simulink model "ThreeLinkCyl"  (Simulink 7.6)
settings: Solver=ode45  StartTime=0.0  StopTime=10.0  RelTol=1e-3
libraries: roblocks x3, simulink x1
settings Model: Creator=mahyar  LastModifiedBy=mahyar

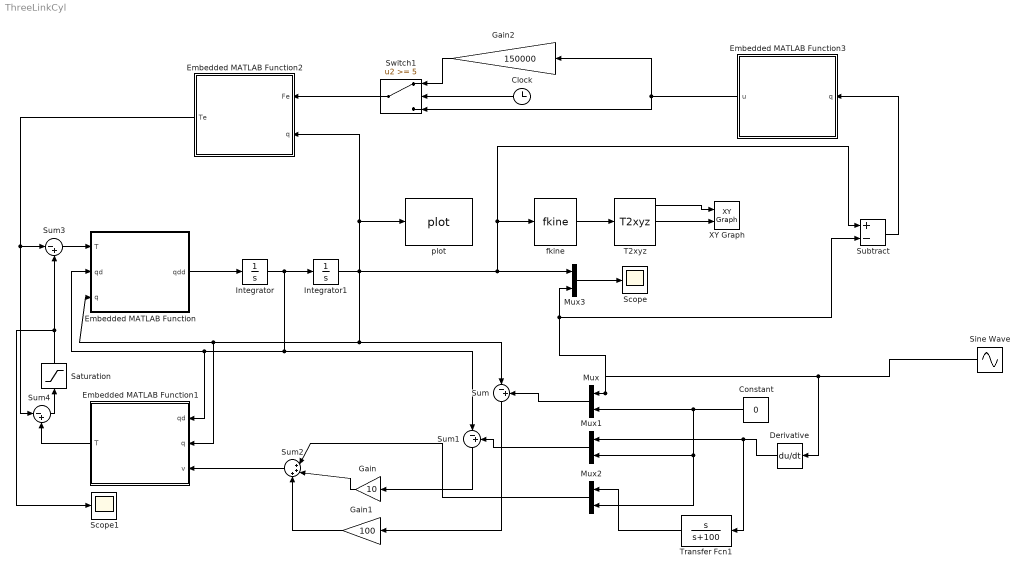
== system ThreeLinkCyl ==
  Clock : Clock
      settings: Decimation=10
  Constant : Constant  Value=0
  Derivative : Derivative
  Embedded MATLAB Function : Stateflow chart  TreatAsAtomicUnit=on
  Embedded MATLAB Function1 : Stateflow chart  TreatAsAtomicUnit=on
  Embedded MATLAB Function2 : Stateflow chart  TreatAsAtomicUnit=on
  Embedded MATLAB Function3 : Stateflow chart  TreatAsAtomicUnit=on
  Gain : Gain  Gain=10
  Gain1 : Gain  Gain=100
  Gain2 : Gain  Gain=150000
  Integrator : Integrator  InitialCondition=[0 0]
  Integrator1 : Integrator  InitialCondition=[0 0]
  Mux{,1..3} (4 alike) : Mux  Inputs=2
  Saturation : Saturate  UpperLimit=85  LowerLimit=-85
  Scope : Scope
      settings: YMin=-1  YMax=1
  Scope1 : Scope
      settings: YMin=-100  YMax=100
  Sine Wave : Sin  SampleTime=0
  Subtract : Sum  Inputs=+-
  Sum{,1,3..4} (4 alike) : Sum  Inputs=|-+
  Sum2 : Sum  Inputs=|+++
  Switch1 : Switch  Threshold=5
  T2xyz : roblocks/T2xyz  SystemSampleTime=-1
  Transfer Fcn1 : TransferFcn  Numerator=[1 0]  Denominator=[1 100]
  XY Graph : simulink/Sinks/XY Graph  SystemSampleTime=-1  xmin=-2  xmax=2  ymin=-2  ymax=2  st=-1
  fkine : roblocks/fkine  SystemSampleTime=-1  robot=tl
  plot : roblocks/plot  SystemSampleTime=-1  robot=tl
  wires:
  Embedded MATLAB Function/1(qdd) -> Integrator/1
  Integrator/1 -> Integrator1/1, Embedded MATLAB Function/2(qd), Embedded MATLAB Function1/1(qd), Sum1/1
  Integrator1/1 -> Embedded MATLAB Function/3(q), Embedded MATLAB Function1/2(q), Sum/1, Mux3/1, fkine/1, Subtract/1, plot/1, Embedded MATLAB Function2/2(q)
  Gain1/1 -> Sum2/3
  Gain/1 -> Sum2/2
  Sum1/1 -> Gain/1
  Sum/1 -> Gain1/1
  Sum2/1 -> Embedded MATLAB Function1/3(v)
  Mux/1 -> Sum/2
  Mux1/1 -> Sum1/2
  Mux2/1 -> Sum2/1
  Derivative/1 -> Mux1/1, Transfer Fcn1/1
  Mux3/1 -> Scope/1
  fkine/1 -> T2xyz/1
  T2xyz/1 -> XY Graph/1
  T2xyz/2 -> XY Graph/2
  Constant/1 -> Mux1/2, Mux2/2, Mux/2
  Embedded MATLAB Function1/1(T) -> Sum4/2
  Sum3/1 -> Embedded MATLAB Function/1(T)
  Subtract/1 -> Embedded MATLAB Function3/1(q)
  Switch1/1 -> Embedded MATLAB Function2/1(Fe)
  Gain2/1 -> Switch1/1
  Embedded MATLAB Function3/1(u) -> Gain2/1, Switch1/3
  Clock/1 -> Switch1/2
  Embedded MATLAB Function2/1(Te) -> Sum3/1, Sum4/1
  Saturation/1 -> Sum3/2, Scope1/1
  Sum4/1 -> Saturation/1
  Transfer Fcn1/1 -> Mux2/1
  Sine Wave/1 -> Mux3/2, Subtract/2, Mux/1, Derivative/1

== matlab function Embedded MATLAB Function1 ==
  data: T output double; qd input double; q input double; v input double
function T = fcn(qd,q,v)

q = [ 0 ; 0 ];
qd = [0 ; 0];

q1 = q(1);
q2 = q(2);

qd1 = qd(1);
qd2 = qd(2);

%**************************************************************************

l1 = 0.35;
l2 = 0.294;

m1=11.17;
m2=6.82;

L1=0.30;
L2=0.18;

I1=1.0;
I2=0.224;

g=0;
%**************************************************************************

d11 = m1*L1^2 + m2*(l1^2 + L2^2 + 2*l1*L2*cos(q2))+I1+I2;
d12 = m2*(L2^2 + l1*L2*cos(q2)) + I2;
d21 = m2*(L2^2 + l1*L2*cos(q2)) + I2;
d22 = m2*L2^2 +I2;

g1 = (m1*L1+m2*l1)*g*cos(q1)+m2*L2*g*cos(q1+q2);
g2 = m2*L2*g*cos(q1+q2);


h = -m2*l1*L2*sin(q2);
c121 = h;
c211 = h;
c221 = h;
c112 = -h;


%**************************************************************************

D = [d11 d12 ; d21 d22];
C = [h*qd2  h*qd2+h*qd1 ; -h*qd1 0];
G = [g1 ; g2];

%**************************************************************************
T = D*v+C*qd+G;

== matlab function Embedded MATLAB Function ==
  data: T input double; qdd output double; qd input double; q input double
function qdd = fcn(T,qd,q)

q = [ 0 ; 0 ];
qd = [0 ; 0];

q1 = q(1);
q2 = q(2);

qd1 = qd(1);
qd2 = qd(2);

t1 = T(1);
t2 = T(2);

%**************************************************************************

l1 = 0.35;
l2 = 0.294;

m1=11.17;
m2=6.82;

L1=0.30;
L2=0.18;

I1=1.0;
I2=0.224;

g=0;
%**************************************************************************

d11 = m1*L1^2 + m2*(l1^2 + L2^2 + 2*l1*L2*cos(q2))+I1+I2;
d12 = m2*(L2^2 + l1*L2*cos(q2)) + I2;
d21 = m2*(L2^2 + l1*L2*cos(q2)) + I2;
d22 = m2*L2^2 +I2;

g1 = (m1*L1+m2*l1)*g*cos(q1)+m2*L2*g*cos(q1+q2);
g2 = m2*L2*g*cos(q1+q2);


h = -m2*l1*L2*sin(q2);
c121 = h;
c211 = h;
c221 = h;
c112 = -h;


%**************************************************************************

D = [d11 d12 ; d21 d22];
C = [h*qd2  h*qd2+h*qd1 ; -h*qd1 0];
G = [g1 ; g2];

%**************************************************************************

qdd= inv(D) * ((-C)*qd+T-G);

== matlab function Embedded MATLAB Function2 ==
  data: Fe input double; Te output double; q input double
function Te = fcn(Fe,q)

a1 = 1;
a2 = 1;
s1 = sin(q(1));
s12 = sin(q(1)+q(2));
c1 = cos(q(1));
c12= cos(q(1)+q(2));

%**************************************************************************

J=[-a1*s1-a2*s12  ,  -a2*s12;
    a1*c1+a2*c12  ,  a2*c12;
    0             ,  0;
    0             ,  0;
    0             ,  0;
    1             ,  1];

%**************************************************************************

Te = J'*Fe;

== matlab function Embedded MATLAB Function3 ==
  data: u output double; q input double
function u = fcn(q)

a1 = 1;
a2 = 1;
s1 = sin(q(1));
s12 = sin(q(1)+q(2));
c1 = cos(q(1));
c12= cos(q(1)+q(2));

%**************************************************************************

J=[-a1*s1-a2*s12  ,  -a2*s12;
    a1*c1+a2*c12  ,  a2*c12;
    0             ,  0;
    0             ,  0;
    0             ,  0;
    1             ,  1];

%**************************************************************************

u = J*q;
